simulink model "Point_Absorber_1D_ESC_K_B_classic_LOG_MM"  (R2019b)
settings: Solver=ode4  StartTime=par.sym.TStart  StopTime=par.sym.TStop  FixedStep=par.sym.max_dt  MaxStep=par.sym.max_dt  RelTol=1e-3
undefined symbols (not defined in the file): a_B, a_K, B_0, B_init, Cdz, density_p, Diam, drag_flag, g, Initial_L, K_0, k_B, K_init, k_K, L, m, mooring_flag, N_delay, par, phase, Pto_flag, R, Sat, Smax, T_tran, volume, w_1_B, w_1_K, w_B, w_K, W_K, w_L_B, w_L_K, wave_flag
libraries: simulink x1
settings Model: Creator=Vitù  LastModifiedBy=User
settings DataIOCC: SaveFormat=Array  SaveOutput=off  SignalLogging=off  DSMLogging=off  ReturnWorkspaceOutputs=off  TimeSaveName=TIME  OutputSaveName=Yout  OutputOption=SpecifiedOutputTimes  OutputTimes=[par.sym.TStart:par.sym.Outputdt:par.sym.TStop]
settings OptimizationCC: ExpressionDepthLimit=2147483647  LifeSpan=inf
settings DebuggingCC: UnderspecifiedInitializationDetection=Classic  MergeDetectMultiDrivingBlocksExec=none  SolverPrmCheckMsg=warning  AllowSymbolicDim=off  StateNameClashWarn=warning  SFUnexpectedBacktrackingDiag=warning  SFNoUnconditionalDefaultTransitionDiag=warning  SFExecutionAtInitializationDiag=none  ArithmeticOperatorsInVariantConditions=warning
settings HardwareCC: ProdBitPerPointer=32  ProdBitPerSizeT=32  ProdBitPerPtrDiffT=32  ProdLargestAtomicFloat=None  ProdIntDivRoundTo=Undefined  ProdEndianess=Unspecified  ProdWordSize=32  ProdHWDeviceType=32-bit Generic
settings ModelReferenceCC: PropagateSignalLabelsOutOfModel=off
settings SFSimCC: SimUseLocalCustomCode=off  CustomCodeUndefinedFunction=UseInterfaceOnly
settings RTWCC: RTWUseLocalCustomCode=off
settings CodeAppCC: StateflowObjectComments=on
settings GRTTargetCC: TargetLangStandard=C89/C90 (ANSI)  GeneratePreprocessorConditionals=Disable all
settings ConfigComp: CovMetricSettings=dw  CovHtmlReporting=on  CovSaveCumulativeToWorkspaceVar=on  CovSaveSingleToWorkspaceVar=on  CovExternalEMLEnable=off  CovSFcnEnable=off
settings SimscapeCC: SimscapeNormalizeSystem=off
settings ConfigurationSet: Description=SimMechanics 2G

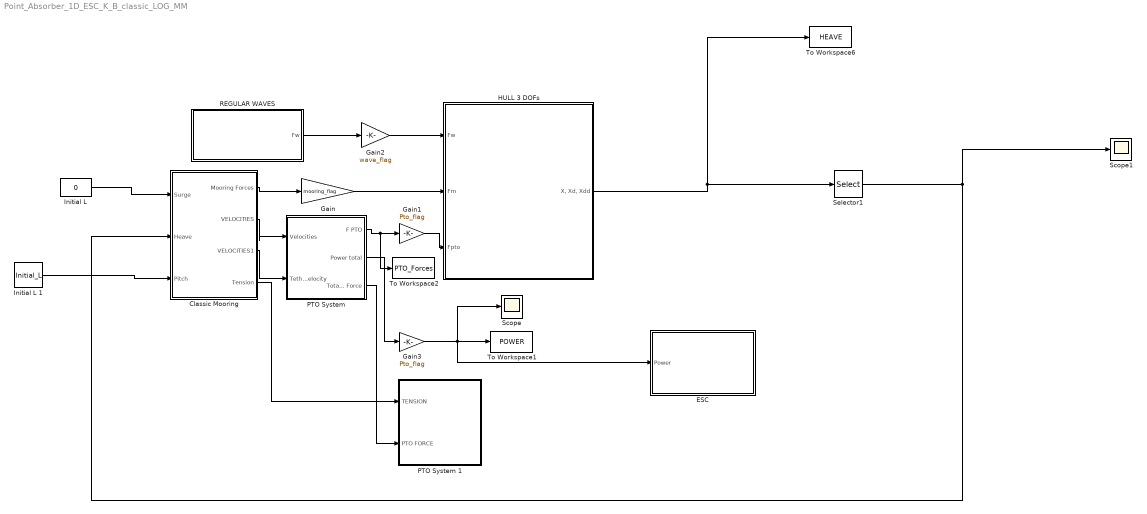
== system Point_Absorber_1D_ESC_K_B_classic_LOG_MM ==
  Classic Mooring : Subsystem
  ESC : Subsystem
  Gain : Gain  Gain=mooring_flag
  Gain1 : Gain  Gain=Pto_flag
  Gain2 : Gain  Gain=wave_flag
  Gain3 : Gain  Gain=Pto_flag
  HULL 3 DOFs : Subsystem
  "Initial L " : Constant  Value=0
  Initial L 1 : Constant  Value=Initial_L
  "PTO System " : Subsystem
  PTO System 1 : Subsystem
  REGULAR WAVES : Subsystem
  Scope : Scope
  Scope1 : Scope
  Selector1 : Selector  InputPortWidth=3  IndexOptions=Index vector (dialog)  Indices=[1]  OutputSizes=1
  To Workspace1 : ToWorkspace  VariableName=POWER  SampleTime=-1
  To Workspace2 : ToWorkspace  VariableName=PTO_Forces  SampleTime=-1
  To Workspace6 : ToWorkspace  VariableName=HEAVE  SampleTime=-1
  wires:
  REGULAR WAVES/1(Fw) -> Gain2/1
  Selector1/1 -> Classic Mooring/2("Heave "), Scope1/1
  "PTO System "/1(F PTO) -> To Workspace2/1, Gain1/1
  Gain2/1 -> HULL 3 DOFs/1(Fw)
  HULL 3 DOFs/1("X, Xd, Xdd") -> Selector1/1, To Workspace6/1
  Gain/1 -> HULL 3 DOFs/2(Fm)
  Gain1/1 -> HULL 3 DOFs/3(Fpto)
  "PTO System "/2(Power total) -> Gain3/1
  Gain3/1 -> ESC/1(Power), Scope/1, To Workspace1/1
  Classic Mooring/1(Mooring Forces) -> Gain/1
  Classic Mooring/2(VELOCITIES) -> "PTO System "/1(Velocities)
  Classic Mooring/3(VELOCITIES1) -> "PTO System "/2(Tether Velocity)
  Classic Mooring/4(Tension) -> PTO System 1/1(TENSION)
  "PTO System "/3("Total PTO Force ") -> PTO System 1/2("PTO FORCE ")
  "Initial L "/1 -> Classic Mooring/1(Surge)
  Initial L 1/1 -> Classic Mooring/3(Pitch)

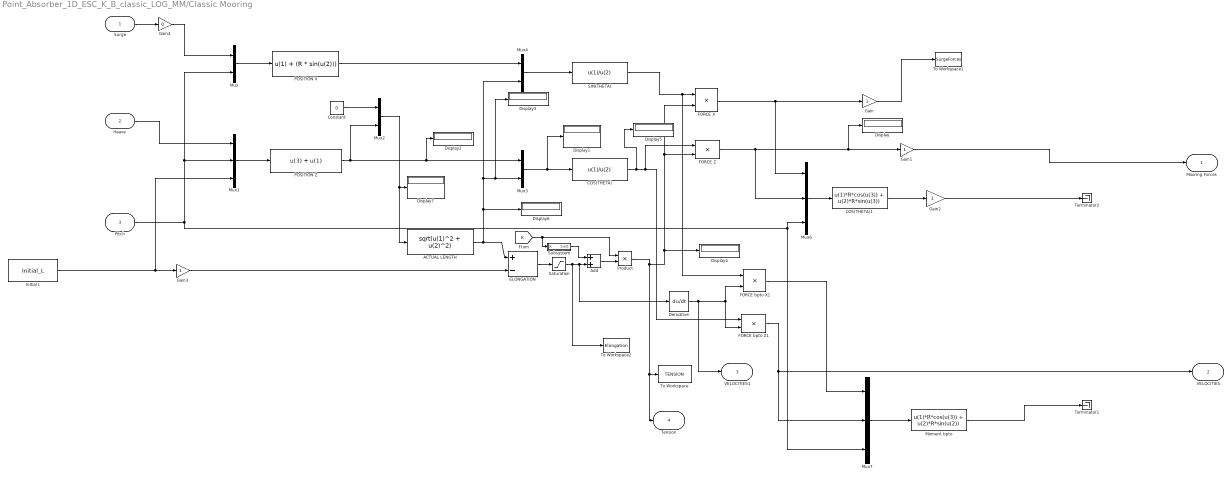
== system Point_Absorber_1D_ESC_K_B_classic_LOG_MM/Classic Mooring ==
  Surge : Inport
  "Heave " : Inport  Port=2
  Pitch : Inport  Port=3
  ACTUAL LENGTH : Fcn  Expr=sqrt(u(1)^2 + u(2)^2)
  Add : Sum
  COS(THETA) : Fcn  Expr=u(1)/u(2)
  COS(THETA)1 : Fcn  Expr=u(1)*R*cos(u(3)) + u(2)*R*sin(u(3))
  Constant : Constant  Value=0
  Derivative : Derivative
  Display{,1..7} (8 alike) : Display
  ELONGATION : Sum  Inputs=+-
  FORCE X : Product
  FORCE Z : Product
  FORCE bpto X1 : Product
  FORCE bpto Z1 : Product
  Gain{,1..3} (4 alike) : Gain
  Gain4 : Gain  Gain=0
  "Initial L " : Constant  Value=Initial_L
  Moment bpto : Fcn  Expr=u(1)*R*cos(u(3)) + u(2)*R*sin(u(2))
  Mux{,2..4} (4 alike) : Mux  Inputs=2
  Mux1 : Mux  Inputs=3
  Mux6 : Mux  Inputs=3
  Mux7 : Mux  Inputs=3
  POSITION X : Fcn  Expr=u(1) + (R * sin(u(2)))
  POSITION Z : Fcn  Expr=u(3) + u(1)
  Product : Product
  SIN(THETA) : Fcn  Expr=u(1)/u(2)
  Saturation : Saturate  UpperLimit=Smax  LowerLimit=-Smax
  Subsystem : Subsystem
  Terminator1 : Terminator
  Terminator2 : Terminator
  To Workspace : ToWorkspace  VariableName=TENSION  SampleTime=-1
  To Workspace1 : ToWorkspace  VariableName=SurgeForces  SampleTime=-1
  To Workspace2 : ToWorkspace  VariableName=Elongation  SampleTime=-1
  Mooring Forces : Outport  VectorParamsAs1DForOutWhenUnconnected=off
  VELOCITIES : Outport  Port=2  VectorParamsAs1DForOutWhenUnconnected=off
  VELOCITIES1 : Outport  Port=3  VectorParamsAs1DForOutWhenUnconnected=off
  Tension : Outport  Port=4  VectorParamsAs1DForOutWhenUnconnected=off
  wires:
  Surge/1 -> Gain4/1
  Mux/1 -> POSITION X/1
  Pitch/1 -> Mux1/2, Mux/2, Mux6/3, Mux7/3
  Mux1/1 -> POSITION Z/1
  "Heave "/1 -> Mux1/1
  POSITION Z/1 -> Display2/1, Mux3/1, Mux2/2
  POSITION X/1 -> Mux4/1
  Mux2/1 -> Display7/1, ACTUAL LENGTH/1
  ELONGATION/1 -> Saturation/1
  Mux4/1 -> SIN(THETA)/1
  Mux3/1 -> Display1/1, COS(THETA)/1
  Product/1 -> Tension/1, To Workspace/1, Display4/1, FORCE Z/2, FORCE X/2
  SIN(THETA)/1 -> FORCE bpto X1/1, FORCE X/1
  COS(THETA)/1 -> Display5/1, FORCE bpto Z1/1, FORCE Z/1
  FORCE Z/1 -> Mux6/2, Display/1, Gain1/1
  COS(THETA)1/1 -> Gain2/1
  Mux6/1 -> COS(THETA)1/1
  Gain1/1 -> Mooring Forces/1
  Derivative/1 -> VELOCITIES1/1, FORCE bpto X1/2, FORCE bpto Z1/2
  FORCE bpto X1/1 -> Mux7/1
  Mux7/1 -> Moment bpto/1
  Moment bpto/1 -> Terminator1/1
  FORCE bpto Z1/1 -> VELOCITIES/1, Mux7/2
  FORCE X/1 -> Mux6/1, Gain/1
  Gain/1 -> To Workspace1/1
  Gain2/1 -> Terminator2/1
  Add/1 -> Product/2
  Subsystem/1(Sinit) -> Add/1
  Saturation/1 -> Add/2, Derivative/1, To Workspace2/1
  Gain3/1 -> ELONGATION/2
  Gain4/1 -> Mux/1
  ACTUAL LENGTH/1 -> ELONGATION/1, Mux3/2, Display3/1, Mux4/2, Display6/1
  Constant/1 -> Mux2/1
  [K] -> Subsystem/1(K), Product/1
  "Initial L "/1 -> Mux1/3, Gain3/1

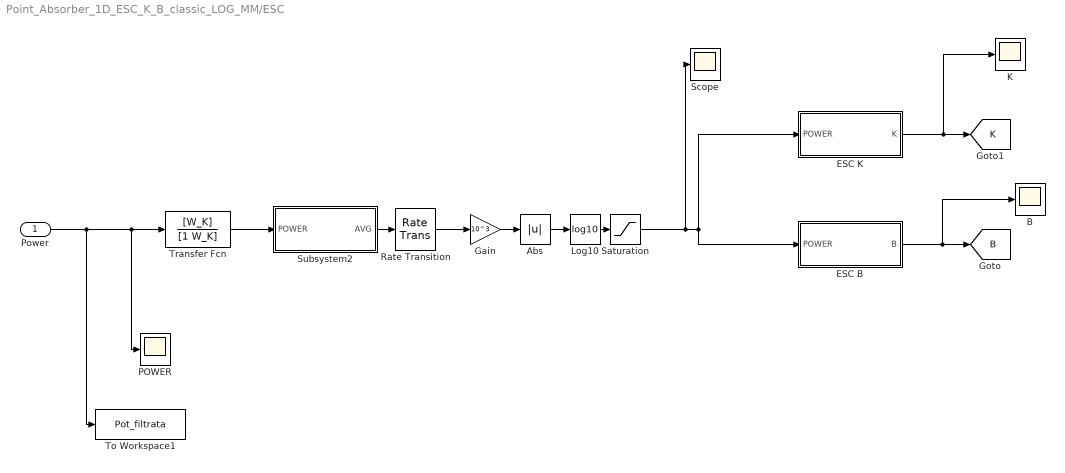
== system Point_Absorber_1D_ESC_K_B_classic_LOG_MM/ESC ==
  Power : Inport
  Abs : Abs
  B : Scope
  ESC B : Subsystem
  ESC K : Subsystem
  Gain : Gain  Gain=10^3
  K : Scope
  Log10 : Math  Operator=log10  SignedPower=off  SaturateOnIntegerOverflow=on
  POWER : Scope
  Rate Transition : RateTransition
  Saturation : Saturate  UpperLimit=inf  LowerLimit=-20
  Scope : Scope
  Subsystem2 : Subsystem
  To Workspace1 : ToWorkspace  VariableName=Pot_filtrata  SampleTime=-1
  Transfer Fcn : TransferFcn  Numerator=[W_K]  Denominator=[1 W_K]
  tag scope: B=global, K=global
  wires:
  Power/1 -> Transfer Fcn/1, POWER/1, To Workspace1/1
  ESC B/1(B) -> B/1, [B]
  ESC K/1(K) -> K/1, [K]
  Subsystem2/1(AVG) -> Rate Transition/1
  Saturation/1 -> Scope/1, ESC B/1(POWER), ESC K/1(POWER)
  Rate Transition/1 -> Gain/1
  Log10/1 -> Saturation/1
  Transfer Fcn/1 -> Subsystem2/1(POWER)
  Abs/1 -> Log10/1
  Gain/1 -> Abs/1

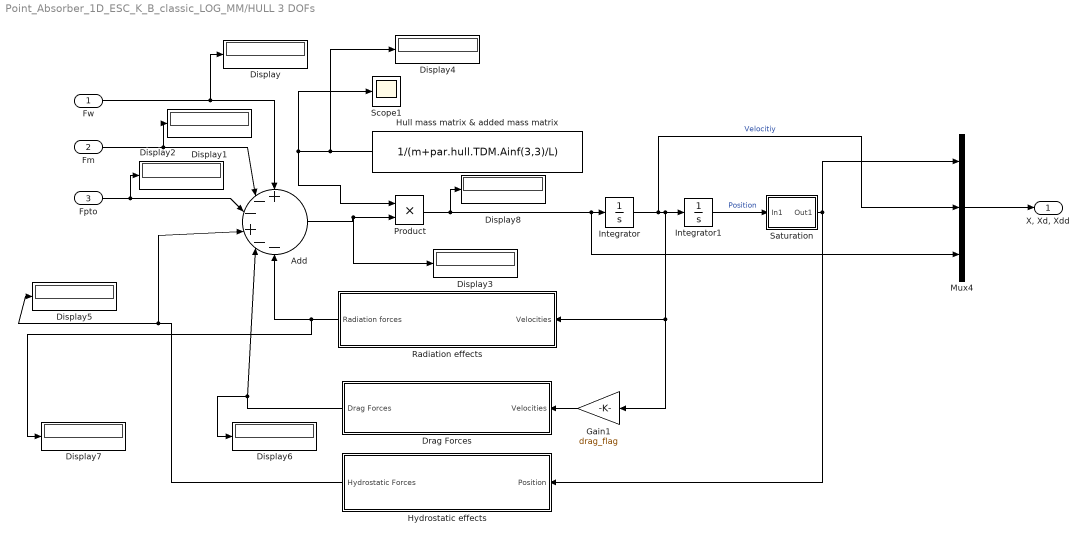
== system Point_Absorber_1D_ESC_K_B_classic_LOG_MM/HULL 3 DOFs ==
  Fw : Inport
  Fm : Inport  Port=2
  Fpto : Inport  Port=3
  Add : Sum  Inputs=+--+--
  Display{,1..8} (9 alike) : Display
  Drag Forces : Subsystem
  Gain1 : Gain  Gain=drag_flag
  Hull mass matrix & added mass matrix : Constant  Value=1/(m+par.hull.TDM.Ainf(3,3)/L)
  Hydrostatic effects : Subsystem
  Integrator : Integrator
  Integrator1 : Integrator
  Mux4 : Mux  Inputs=3
  Product : Product
  Radiation effects : Subsystem
  Saturation : Subsystem
  Scope1 : Scope
  "X, Xd, Xdd" : Outport  VectorParamsAs1DForOutWhenUnconnected=off
  wires:
  Integrator/1 -> Integrator1/1, Gain1/1, Radiation effects/1(Velocities), Mux4/2  "Velocitiy"
  Integrator1/1 -> Saturation/1(In1)  "Position"
  Hull mass matrix & added mass matrix/1 -> Display4/1, Product/1, Scope1/1
  Fw/1 -> Display/1, Add/1
  Product/1 -> Display8/1, Mux4/3, Integrator/1
  Mux4/1 -> "X, Xd, Xdd"/1
  Fm/1 -> Display1/1, Add/2
  Gain1/1 -> Drag Forces/1(Velocities)
  Fpto/1 -> Display2/1, Add/3
  Radiation effects/1(Radiation forces) -> Display7/1, Add/6
  Hydrostatic effects/1("Hydrostatic Forces ") -> Add/4, Display5/1
  Add/1 -> Display3/1, Product/2
  Saturation/1(Out1) -> Mux4/1, Hydrostatic effects/1(Position)
  Drag Forces/1(Drag Forces) -> Add/5, Display6/1

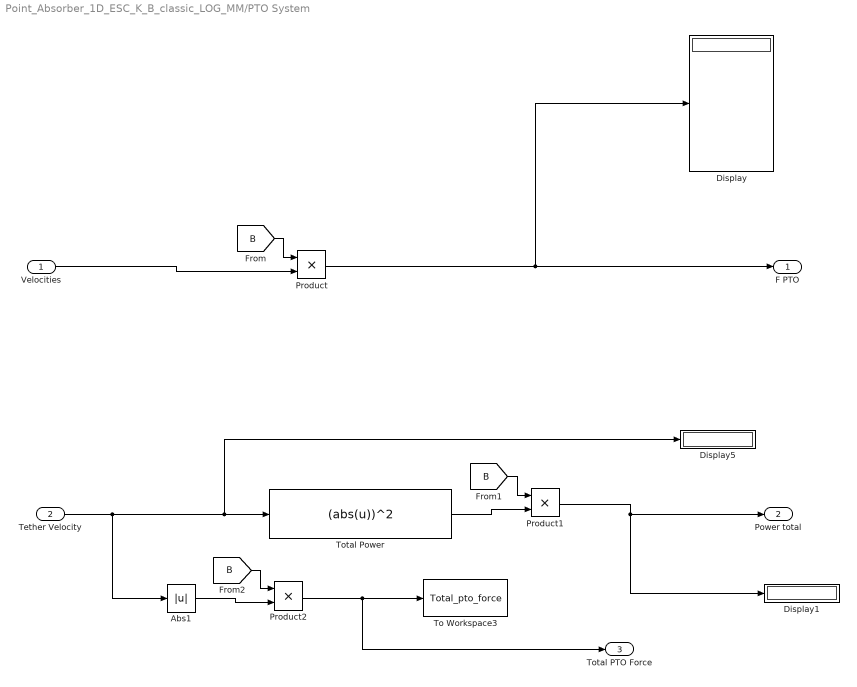
== system Point_Absorber_1D_ESC_K_B_classic_LOG_MM/PTO System  ==
  Velocities : Inport
  Tether Velocity : Inport  Port=2
  Abs1 : Abs  ZeroCross=off
  Display : Display
  Display1 : Display
  Display5 : Display
  Product : Product
  Product1 : Product
  Product2 : Product
  To Workspace3 : ToWorkspace  VariableName=Total_pto_force  SampleTime=-1
  Total Power : Fcn  Expr=(abs(u))^2
  F PTO : Outport  VectorParamsAs1DForOutWhenUnconnected=off
  Power total : Outport  Port=2  VectorParamsAs1DForOutWhenUnconnected=off
  "Total PTO Force " : Outport  Port=3  VectorParamsAs1DForOutWhenUnconnected=off
  wires:
  Product/1 -> Display/1, F PTO/1
  Product1/1 -> Display1/1, Power total/1
  Velocities/1 -> Product/2
  Abs1/1 -> Product2/2
  Product2/1 -> "Total PTO Force "/1, To Workspace3/1
  Tether Velocity/1 -> Abs1/1, Total Power/1, Display5/1
  [B] -> Product/1
  [B] -> Product1/1
  Total Power/1 -> Product1/2
  [B] -> Product2/1

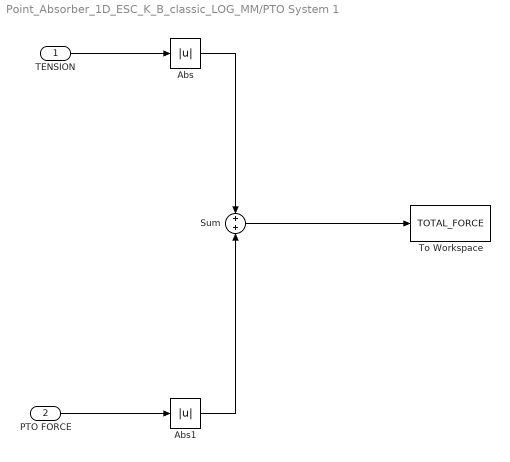
== system Point_Absorber_1D_ESC_K_B_classic_LOG_MM/PTO System 1 ==
  TENSION : Inport
  "PTO FORCE " : Inport  Port=2
  Abs : Abs  ZeroCross=off
  Abs1 : Abs  ZeroCross=off
  Sum : Sum
  To Workspace : ToWorkspace  VariableName=TOTAL_FORCE  SampleTime=-1
  wires:
  TENSION/1 -> Abs/1
  "PTO FORCE "/1 -> Abs1/1
  Abs/1 -> Sum/1
  Abs1/1 -> Sum/2
  Sum/1 -> To Workspace/1

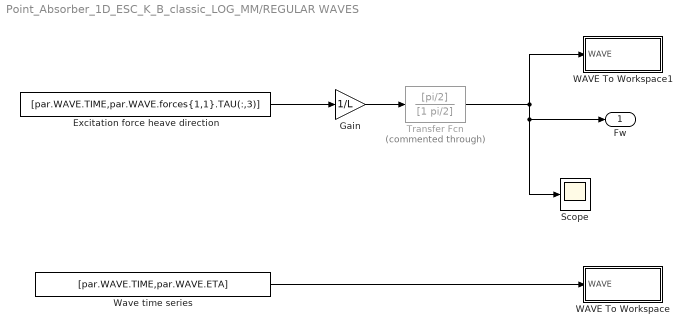
== system Point_Absorber_1D_ESC_K_B_classic_LOG_MM/REGULAR WAVES ==
  Excitation force heave direction : FromWorkspace  VariableName=[par.WAVE.TIME,par.WAVE.forces{1,1}.TAU(:,3)]  SampleTime=0
  Gain : Gain  Gain=1/L
  Scope : Scope
  Transfer Fcn : TransferFcn  Commented=through  Numerator=[pi/2]  Denominator=[1 pi/2]
  WAVE To Workspace : Subsystem
  WAVE To Workspace1 : Subsystem
  Wave time series : FromWorkspace  VariableName=[par.WAVE.TIME,par.WAVE.ETA]  SampleTime=0
  Fw : Outport  VectorParamsAs1DForOutWhenUnconnected=off
  wires:
  Wave time series/1 -> WAVE To Workspace/1(WAVE)
  Excitation force heave direction/1 -> Gain/1
  Gain/1 -> Transfer Fcn/1
  Transfer Fcn/1 -> Fw/1, Scope/1, WAVE To Workspace1/1(WAVE)

== system Point_Absorber_1D_ESC_K_B_classic_LOG_MM/Classic Mooring/Subsystem ==
  K : Inport
  Constant : Constant  Value=(density_p*g*volume - m*g)
  Divide : Product  Inputs=*/
  Sinit : Outport
  wires:
  Constant/1 -> Divide/1
  K/1 -> Divide/2
  Divide/1 -> Sinit/1

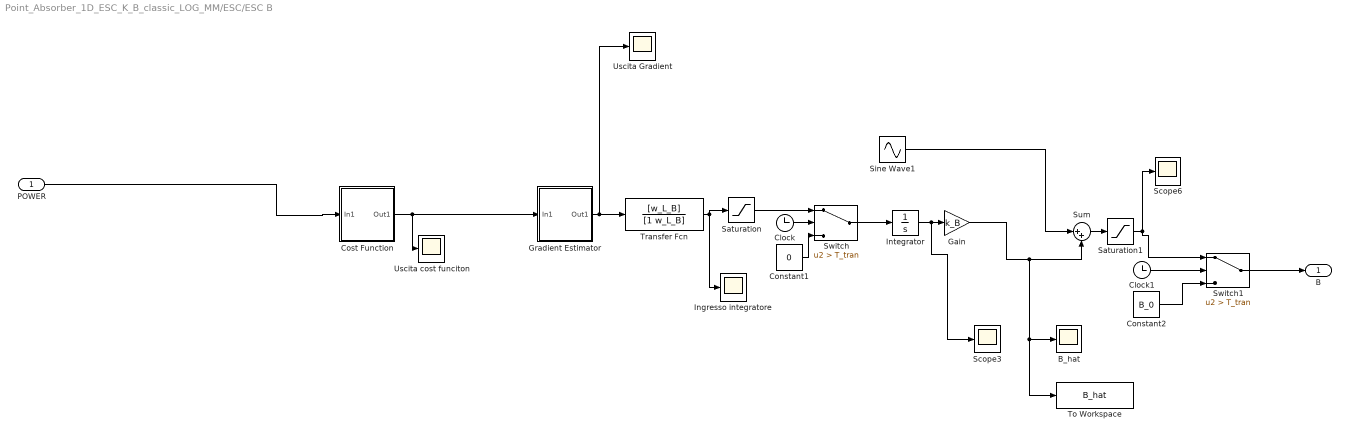
== system Point_Absorber_1D_ESC_K_B_classic_LOG_MM/ESC/ESC B ==
  POWER : Inport
  B_hat : Scope
  Clock : Clock
  Clock1 : Clock
  Constant1 : Constant  Value=0
  Constant2 : Constant  Value=B_0
  Cost Function : Subsystem
  Gain : Gain  Gain=k_B
  Gradient Estimator : Subsystem
  Ingresso integratore : Scope
  Integrator : Integrator  InitialCondition=B_init
  Saturation : Saturate  UpperLimit=Sat  LowerLimit=-Sat
  Saturation1 : Saturate  UpperLimit=inf  LowerLimit=0.1
  Scope3 : Scope
  Scope6 : Scope
  Sine Wave1 : Sin  Amplitude=a_B  Frequency=w_B  SampleTime=0
  Sum : Sum  Inputs=|++
  Switch : Switch  Criteria=u2 > Threshold  Threshold=T_tran
  Switch1 : Switch  Criteria=u2 > Threshold  Threshold=T_tran
  To Workspace : ToWorkspace  VariableName=B_hat  SampleTime=-1
  Transfer Fcn : TransferFcn  Numerator=[w_L_B]  Denominator=[1 w_L_B]
  Uscita Gradient : Scope
  Uscita cost funciton : Scope
  B : Outport
  wires:
  Sine Wave1/1 -> Sum/1
  Gain/1 -> Sum/2, B_hat/1, To Workspace/1
  Constant2/1 -> Switch1/3
  Gradient Estimator/1(Out1) -> Transfer Fcn/1, Uscita Gradient/1
  Transfer Fcn/1 -> Saturation/1, Ingresso integratore/1
  POWER/1 -> Cost Function/1(In1)
  Cost Function/1(Out1) -> Uscita cost funciton/1, Gradient Estimator/1(In1)
  Integrator/1 -> Scope3/1, Gain/1
  Sum/1 -> Saturation1/1
  Clock1/1 -> Switch1/2
  Switch1/1 -> B/1
  Constant1/1 -> Switch/3
  Clock/1 -> Switch/2
  Switch/1 -> Integrator/1
  Saturation/1 -> Switch/1
  Saturation1/1 -> Switch1/1, Scope6/1

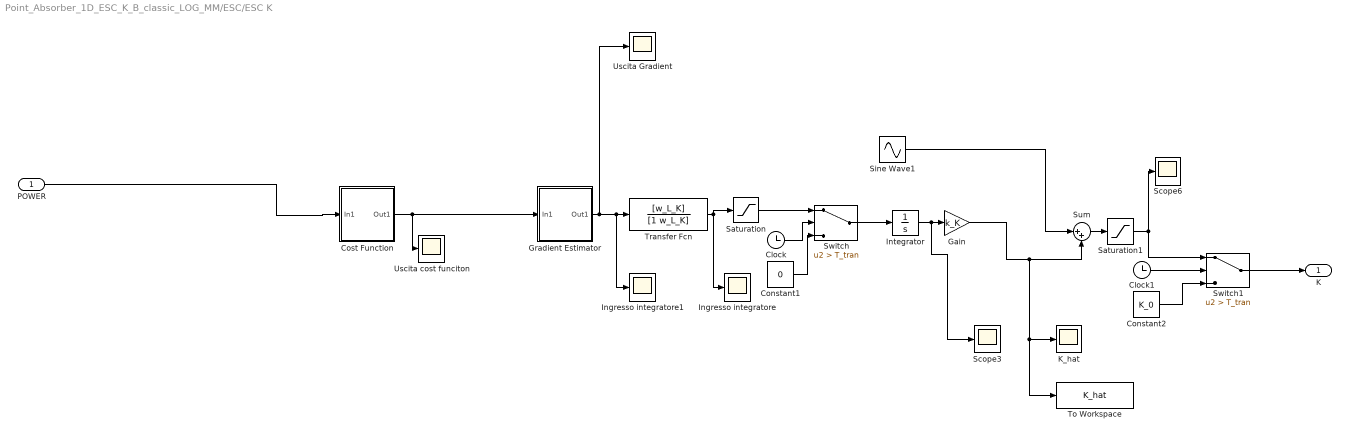
== system Point_Absorber_1D_ESC_K_B_classic_LOG_MM/ESC/ESC K ==
  POWER : Inport
  Clock : Clock
  Clock1 : Clock
  Constant1 : Constant  Value=0
  Constant2 : Constant  Value=K_0
  Cost Function : Subsystem
  Gain : Gain  Gain=k_K
  Gradient Estimator : Subsystem
  Ingresso integratore : Scope
  Ingresso integratore1 : Scope
  Integrator : Integrator  InitialCondition=K_init
  K_hat : Scope
  Saturation : Saturate  UpperLimit=Sat  LowerLimit=-Sat
  Saturation1 : Saturate  UpperLimit=inf  LowerLimit=0.1
  Scope3 : Scope
  Scope6 : Scope
  Sine Wave1 : Sin  Amplitude=a_K  Frequency=w_K  SampleTime=0
  Sum : Sum  Inputs=|++
  Switch : Switch  Criteria=u2 > Threshold  Threshold=T_tran
  Switch1 : Switch  Criteria=u2 > Threshold  Threshold=T_tran
  To Workspace : ToWorkspace  VariableName=K_hat  SampleTime=-1
  Transfer Fcn : TransferFcn  Numerator=[w_L_K]  Denominator=[1 w_L_K]
  Uscita Gradient : Scope
  Uscita cost funciton : Scope
  K : Outport
  wires:
  Switch1/1 -> K/1
  Clock1/1 -> Switch1/2
  Sum/1 -> Saturation1/1
  Integrator/1 -> Gain/1, Scope3/1
  Cost Function/1(Out1) -> Gradient Estimator/1(In1), Uscita cost funciton/1
  POWER/1 -> Cost Function/1(In1)
  Transfer Fcn/1 -> Ingresso integratore/1, Saturation/1
  Gradient Estimator/1(Out1) -> Uscita Gradient/1, Transfer Fcn/1, Ingresso integratore1/1
  Constant2/1 -> Switch1/3
  Gain/1 -> To Workspace/1, K_hat/1, Sum/2
  Sine Wave1/1 -> Sum/1
  Clock/1 -> Switch/2
  Constant1/1 -> Switch/3
  Switch/1 -> Integrator/1
  Saturation/1 -> Switch/1
  Saturation1/1 -> Scope6/1, Switch1/1

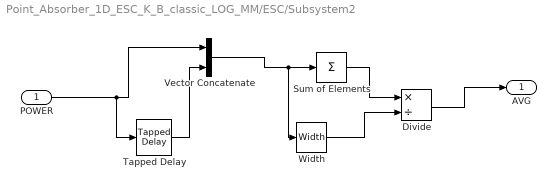
== system Point_Absorber_1D_ESC_K_B_classic_LOG_MM/ESC/Subsystem2 ==
  POWER : Inport
  Divide : Product  Inputs=*/
  Sum of Elements : Sum  Inputs=+
  Tapped Delay : simulink/Discrete/Tapped Delay  vinit=0  samptime=-1  NumDelays=N_delay  DelayOrder=Oldest  includeCurrent=off
  Vector Concatenate : Concatenate
  Width : Width
  AVG : Outport
  wires:
  POWER/1 -> Tapped Delay/1, Vector Concatenate/1
  Tapped Delay/1 -> Vector Concatenate/2
  Vector Concatenate/1 -> Width/1, Sum of Elements/1
  Sum of Elements/1 -> Divide/1
  Width/1 -> Divide/2
  Divide/1 -> AVG/1

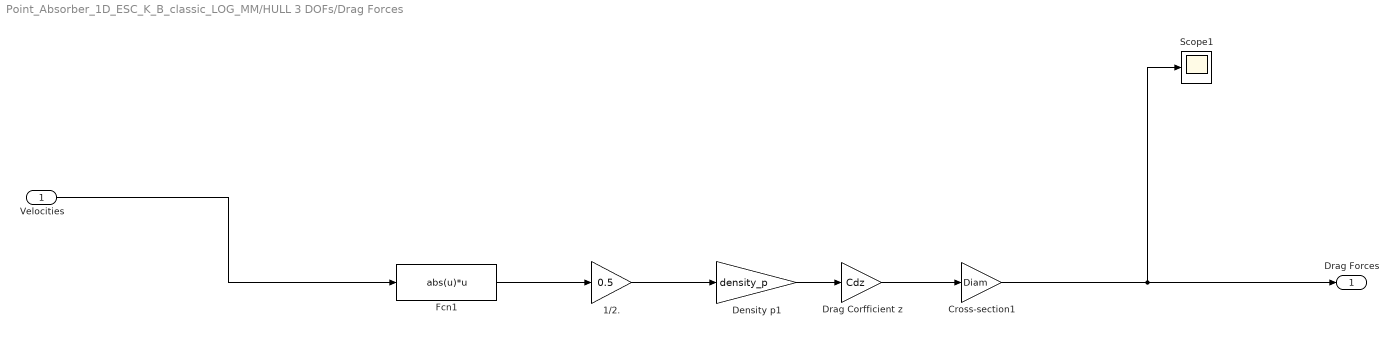
== system Point_Absorber_1D_ESC_K_B_classic_LOG_MM/HULL 3 DOFs/Drag Forces ==
  Velocities : Inport
  1/2. : Gain  Gain=0.5
  Cross-section1 : Gain  Gain=Diam
  Density p1 : Gain  Gain=density_p
  Drag Corfficient z : Gain  Gain=Cdz
  Fcn1 : Fcn  Expr=abs(u)*u
  Scope1 : Scope
  Drag Forces : Outport  VectorParamsAs1DForOutWhenUnconnected=off
  wires:
  Velocities/1 -> Fcn1/1
  Fcn1/1 -> 1/2./1
  1/2./1 -> Density p1/1
  Density p1/1 -> Drag Corfficient z/1
  Drag Corfficient z/1 -> Cross-section1/1
  Cross-section1/1 -> Drag Forces/1, Scope1/1

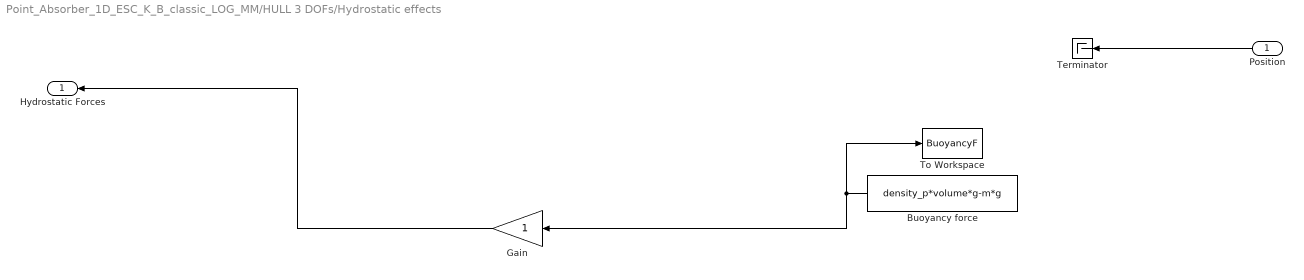
== system Point_Absorber_1D_ESC_K_B_classic_LOG_MM/HULL 3 DOFs/Hydrostatic effects ==
  Position : Inport
  Buoyancy force : Constant  Value=density_p*volume*g-m*g
  Gain : Gain
  Terminator : Terminator
  To Workspace : ToWorkspace  VariableName=BuoyancyF  SampleTime=-1
  "Hydrostatic Forces " : Outport  VectorParamsAs1DForOutWhenUnconnected=off
  wires:
  Gain/1 -> "Hydrostatic Forces "/1
  Buoyancy force/1 -> Gain/1, To Workspace/1
  Position/1 -> Terminator/1

== system Point_Absorber_1D_ESC_K_B_classic_LOG_MM/HULL 3 DOFs/Radiation effects ==
  note: Heave
  Velocities : Inport
  Gain : Gain  Gain=1/L
  State-Space1 : StateSpace  A=par.hull.TDM.z.Ass  B=par.hull.TDM.z.Bss  C=par.hull.TDM.z.Css  D=par.hull.TDM.z.Dss  InitialCondition=0
  Radiation forces : Outport  VectorParamsAs1DForOutWhenUnconnected=off
  wires:
  Velocities/1 -> State-Space1/1
  State-Space1/1 -> Gain/1
  Gain/1 -> Radiation forces/1

== system Point_Absorber_1D_ESC_K_B_classic_LOG_MM/HULL 3 DOFs/Saturation ==
  In1 : Inport
  Saturation2 : Saturate  UpperLimit=Smax  LowerLimit=-Smax
  Out1 : Outport  VectorParamsAs1DForOutWhenUnconnected=off
  wires:
  Saturation2/1 -> Out1/1
  In1/1 -> Saturation2/1

== system Point_Absorber_1D_ESC_K_B_classic_LOG_MM/REGULAR WAVES/WAVE To Workspace ==
  WAVE : Inport
  WAVE Save : ToWorkspace  VariableName=WAVE  SampleTime=-1
  wires:
  WAVE/1 -> WAVE Save/1

== system Point_Absorber_1D_ESC_K_B_classic_LOG_MM/REGULAR WAVES/WAVE To Workspace1 ==
  WAVE : Inport
  WAVEFORCES To Workspace : ToWorkspace  VariableName=WAVEFORCES  SampleTime=-1
  wires:
  WAVE/1 -> WAVEFORCES To Workspace/1

== system Point_Absorber_1D_ESC_K_B_classic_LOG_MM/ESC/ESC B/Cost Function ==
  In1 : Inport
  Ampiezza1 : TransferFcn  Numerator=[1 0]  Denominator=[1 w_1_B]
  Scope7 : Scope
  Out1 : Outport
  wires:
  In1/1 -> Scope7/1, Ampiezza1/1
  Ampiezza1/1 -> Out1/1

== system Point_Absorber_1D_ESC_K_B_classic_LOG_MM/ESC/ESC B/Gradient Estimator ==
  In1 : Inport
  Product : Product
  Scope10 : Scope
  Scope8 : Scope
  Sine Wave : Sin  Frequency=w_B  Phase=phase  SampleTime=0
  Out1 : Outport
  wires:
  In1/1 -> Scope8/1, Product/2, Scope10/1
  Sine Wave/1 -> Product/1
  Product/1 -> Out1/1

== system Point_Absorber_1D_ESC_K_B_classic_LOG_MM/ESC/ESC K/Cost Function ==
  In1 : Inport
  Ampiezza1 : TransferFcn  Numerator=[1 0]  Denominator=[1 w_1_K]
  Scope7 : Scope
  Out1 : Outport
  wires:
  Ampiezza1/1 -> Out1/1
  In1/1 -> Ampiezza1/1, Scope7/1

== system Point_Absorber_1D_ESC_K_B_classic_LOG_MM/ESC/ESC K/Gradient Estimator ==
  In1 : Inport
  Product : Product
  Scope10 : Scope
  Scope8 : Scope
  Sine Wave : Sin  Frequency=w_K  Phase=phase  SampleTime=0
  Out1 : Outport
  wires:
  Product/1 -> Out1/1
  Sine Wave/1 -> Product/1
  In1/1 -> Scope10/1, Product/2, Scope8/1
